simulink model "model6"  (R2022a)
settings: Solver=FixedStepAuto  StartTime=0.0  StopTime=200  FixedStep=1  RelTol=1e-3
values from neighbouring files (symbols this model uses):
  testMap = [0  0  0; 0  99  0; 0  0  0]    [aufgabe2.mat]
settings Model: Creator=JadKHaddad  LastModifiedBy=JadKHaddad

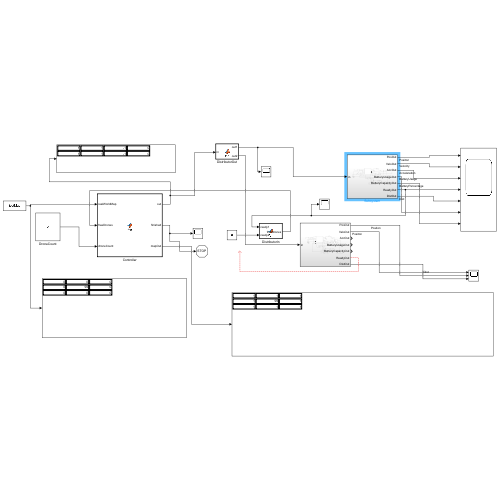
[thumbnail: Simulink's stored preview of the top-level diagram]
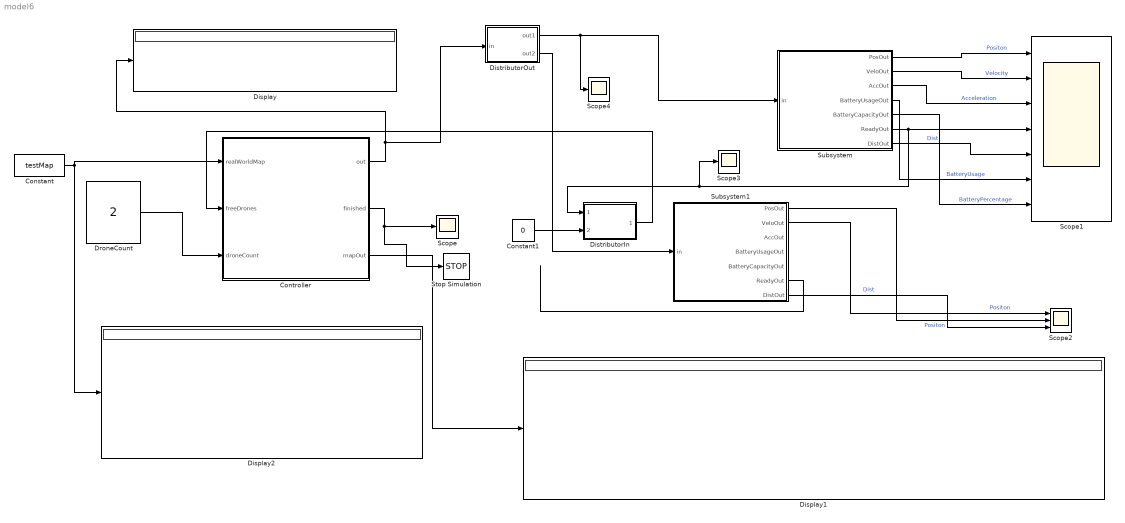
== system model6 ==
  Constant : Constant  Value=testMap  VectorParams1D=off
  Constant1 : Constant  Value=0
  Controller : MATLAB Function  TreatAsAtomicUnit=on
  Display : Display
  Display1 : Display
  Display2 : Display
  DistributorIn : MATLAB Function  TreatAsAtomicUnit=on
  DistributorOut : MATLAB Function  TreatAsAtomicUnit=on
  DroneCount : Constant  Value=2
  Scope : Scope
  Scope1 : Scope  NumInputPorts=7
  Scope2 : Scope  NumInputPorts=3
  Scope3 : Scope
  Scope4 : Scope
  Stop Simulation : Stop
  Subsystem : Subsystem
  Subsystem1 : Subsystem
  wires:
  Subsystem/3(AccOut) -> Scope1/3  "Acceleration"
  Subsystem/1(PosOut) -> Scope1/1  "Positon"
  Subsystem/4(BatteryUsageOut) -> Scope1/6  "BatteryUsage"
  Subsystem/2(VeloOut) -> Scope1/2  "Velocity"
  Subsystem/5(BatteryCapacityOut) -> Scope1/7  "BatteryPercentage"
  Subsystem/6(ReadyOut) -> Scope3/1, DistributorIn/1(ready1), Scope1/4
  Subsystem/7(DistOut) -> Scope1/5  "Dist"
  Controller/2(finished) -> Stop Simulation/1, Scope/1
  Constant/1 -> Display2/1, Controller/1(realWorldMap)
  DroneCount/1 -> Controller/3(droneCount)
  Controller/1(out) -> DistributorOut/1(in), Display/1
  DistributorIn/1(freeDrones) -> Controller/2(freeDrones)
  DistributorOut/1(out1) -> Scope4/1, Subsystem/1(in)
  Controller/3(mapOut) -> Display1/1
  DistributorOut/2(out2) -> Subsystem1/1(in)
  Subsystem1/1(PosOut) -> Scope2/2  "Positon"
  Subsystem1/6(ReadyOut) -> ?
  Subsystem1/7(DistOut) -> Scope2/3  "Dist"
  Subsystem1/2(VeloOut) -> Scope2/1  "Positon"
  Constant1/1 -> DistributorIn/2(ready2)

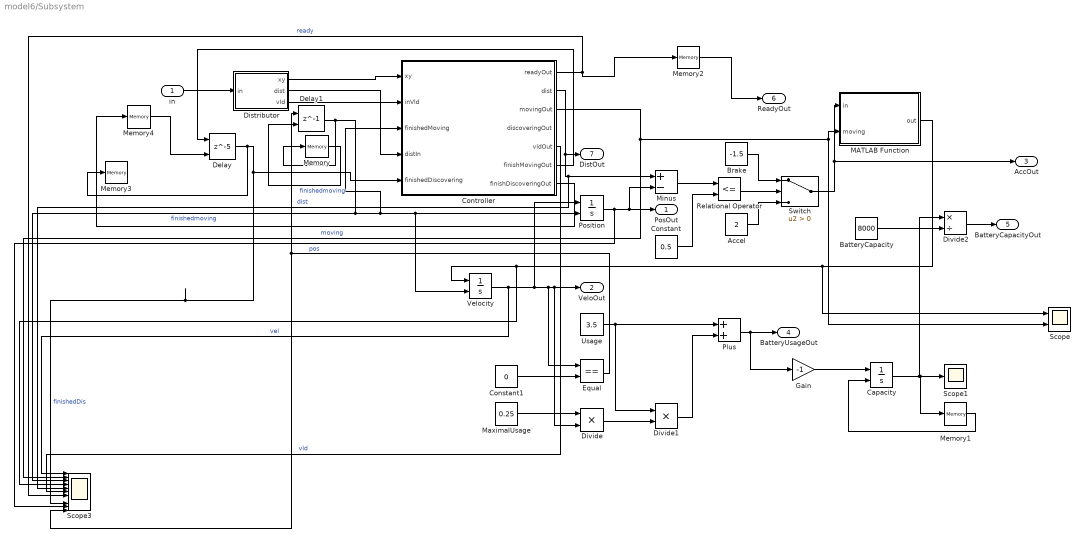
== system model6/Subsystem ==
  in : Inport
  Accel : Constant  Value=2
  BatteryCapacity : Constant  Value=8000
  Brake : Constant  Value=-1.5
  Capacity : Integrator  ExternalReset=rising  InitialCondition=8000  LowerSaturationLimit=0
  Constant : Constant  Value=0.5
  Constant1 : Constant  Value=0
  Controller : MATLAB Function  TreatAsAtomicUnit=on
  Delay : Delay  DelayLength=5  InitialCondition=0  ExternalReset=Rising
      settings: InputPortMap=u0,r5
  Delay1 : Delay  DelayLength=1  ExternalReset=Rising
      settings: InputPortMap=u0,r5
  Distributor : MATLAB Function  TreatAsAtomicUnit=on
  Divide : Product  Inputs=**  RndMeth=Round
  Divide1 : Product  Inputs=**
  Divide2 : Product  Inputs=*/
  Equal : RelationalOperator  Operator===  OutDataTypeStr=boolean  RndMeth=Simplest  InputSameDT=off
  Gain : Gain  Gain=-1
  MATLAB Function : MATLAB Function  TreatAsAtomicUnit=on
  MaximalUsage : Constant  Value=0.25
  Memory : Memory  InheritSampleTime=on
  Memory{1..4} (4 alike) : Memory
  Minus : Sum  Inputs=+-
  Plus : Sum
  Position : Integrator  ExternalReset=rising
  Relational Operator : RelationalOperator  Operator=<=  OutDataTypeStr=boolean  RndMeth=Simplest  InputSameDT=off
  Scope : Scope  NumInputPorts=2
  Scope1 : Scope
  Scope3 : Scope  NumInputPorts=11
  Switch : Switch  Criteria=u2 > Threshold  SaturateOnIntegerOverflow=off  InputSameDT=off
  Usage : Constant  Value=3.5
  Velocity : Integrator  ExternalReset=rising  LimitOutput=on  UpperSaturationLimit=1  LowerSaturationLimit=0
  PosOut : Outport
  VeloOut : Outport  Port=2
  AccOut : Outport  Port=3
  BatteryUsageOut : Outport  Port=4
  BatteryCapacityOut : Outport  Port=5
  ReadyOut : Outport  Port=6
  DistOut : Outport  Port=7
  wires:
  Controller/1(readyOut) -> Memory2/1, Scope3/7  "ready"
  Distributor/1(xy) -> Controller/1(xy)
  Distributor/3(vld) -> Controller/2(inVld)
  Switch/1 -> MATLAB Function/1(in), AccOut/1
  Plus/1 -> Gain/1, BatteryUsageOut/1
  Accel/1 -> Switch/3
  Divide2/1 -> BatteryCapacityOut/1
  Divide/1 -> Divide1/2
  Memory1/1 -> Capacity/2
  Distributor/2(dist) -> Controller/4(distIn)
  Usage/1 -> Plus/1, Divide1/1
  BatteryCapacity/1 -> Divide2/2
  Capacity/1 -> Memory1/1, Scope1/1, Divide2/1
  Gain/1 -> Capacity/1
  Divide1/1 -> Plus/2
  Minus/1 -> Relational Operator/1
  Position/1 -> Scope3/10, Minus/2, PosOut/1  "pos"
  Brake/1 -> Switch/1
  Constant1/1 -> Equal/2
  Relational Operator/1 -> Switch/2
  MaximalUsage/1 -> Divide/1
  Constant/1 -> Relational Operator/2
  Controller/2(dist) -> Minus/1, Scope3/5, DistOut/1  "dist"
  Velocity/1 -> Scope3/1, VeloOut/1, Divide/2, Equal/1, Position/1  "vel"
  Delay1/1 -> Memory/1, Scope3/3, Controller/3(finishedMoving), Velocity/2, Position/2  "finishedmoving"
  in/1 -> Distributor/1(in)
  Memory2/1 -> ReadyOut/1
  MATLAB Function/1(out) -> Scope/1, Scope3/4, Velocity/1
  Equal/1 -> Delay1/1, Scope3/11
  Delay/1 -> Memory3/1, Controller/5(finishedDiscovering), Scope3/9  "finishedDis"
  Controller/3(movingOut) -> Scope3/2, MATLAB Function/2(moving), Scope/2  "moving"
  Controller/5(vldOut) -> Scope3/6  "vld"
  Memory/1 -> Delay1/2  "finishedmoving"
  Controller/7(finishDiscoveringOut) -> Memory4/1
  Memory4/1 -> Delay/2
  Controller/6(finishMovingOut) -> Delay/1

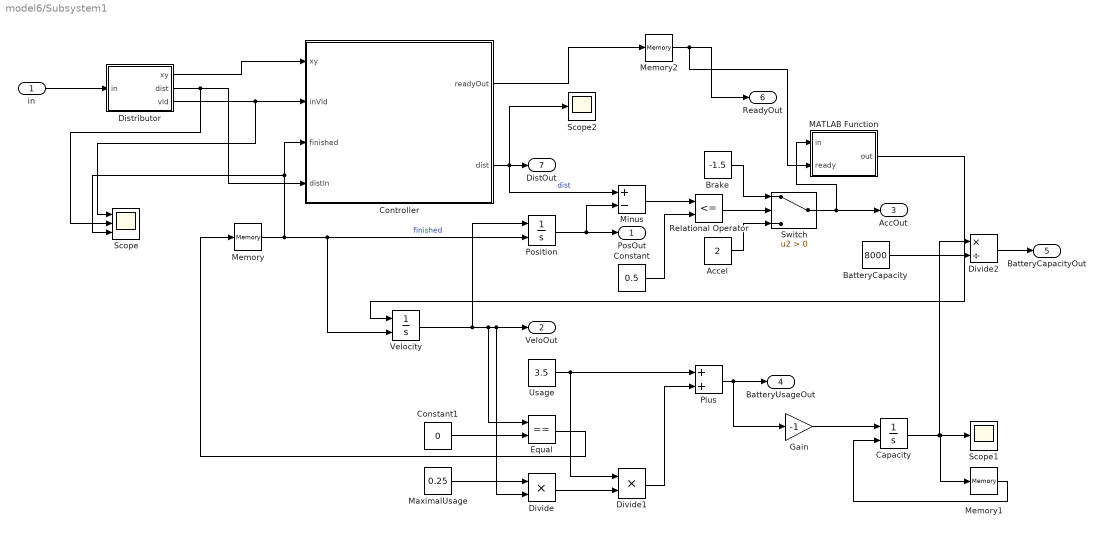
== system model6/Subsystem1 ==
  in : Inport
  Accel : Constant  Value=2
  BatteryCapacity : Constant  Value=8000
  Brake : Constant  Value=-1.5
  Capacity : Integrator  ExternalReset=rising  InitialCondition=8000  LowerSaturationLimit=0
  Constant : Constant  Value=0.5
  Constant1 : Constant  Value=0
  Controller : MATLAB Function  TreatAsAtomicUnit=on
  Distributor : MATLAB Function  TreatAsAtomicUnit=on
  Divide : Product  Inputs=**  RndMeth=Round
  Divide1 : Product  Inputs=**
  Divide2 : Product  Inputs=*/
  Equal : RelationalOperator  Operator===  OutDataTypeStr=boolean  RndMeth=Simplest  InputSameDT=off
  Gain : Gain  Gain=-1
  MATLAB Function : MATLAB Function  TreatAsAtomicUnit=on
  MaximalUsage : Constant  Value=0.25
  Memory : Memory
  Memory1 : Memory
  Memory2 : Memory
  Minus : Sum  Inputs=+-
  Plus : Sum
  Position : Integrator  ExternalReset=rising
  Relational Operator : RelationalOperator  Operator=<=  OutDataTypeStr=boolean  RndMeth=Simplest  InputSameDT=off
  Scope : Scope  NumInputPorts=3
  Scope1 : Scope
  Scope2 : Scope
  Switch : Switch  Criteria=u2 > Threshold  SaturateOnIntegerOverflow=off  InputSameDT=off
  Usage : Constant  Value=3.5
  Velocity : Integrator  ExternalReset=rising  LimitOutput=on  UpperSaturationLimit=1  LowerSaturationLimit=0
  PosOut : Outport
  VeloOut : Outport  Port=2
  AccOut : Outport  Port=3
  BatteryUsageOut : Outport  Port=4
  BatteryCapacityOut : Outport  Port=5
  ReadyOut : Outport  Port=6
  DistOut : Outport  Port=7
  wires:
  Controller/1(readyOut) -> Memory2/1
  Distributor/1(xy) -> Controller/1(xy)
  Distributor/3(vld) -> Scope/1, Controller/2(inVld)
  Switch/1 -> MATLAB Function/1(in), AccOut/1
  Plus/1 -> Gain/1, BatteryUsageOut/1
  Accel/1 -> Switch/3
  Divide2/1 -> BatteryCapacityOut/1
  Divide/1 -> Divide1/2
  Memory1/1 -> Capacity/2
  Distributor/2(dist) -> Scope/2, Controller/4(distIn)
  Usage/1 -> Plus/1, Divide1/1
  BatteryCapacity/1 -> Divide2/2
  Capacity/1 -> Memory1/1, Scope1/1, Divide2/1
  Gain/1 -> Capacity/1
  Divide1/1 -> Plus/2
  Minus/1 -> Relational Operator/1
  Position/1 -> Minus/2, PosOut/1
  Equal/1 -> Memory/1
  Brake/1 -> Switch/1
  Constant1/1 -> Equal/2
  Relational Operator/1 -> Switch/2
  MaximalUsage/1 -> Divide/1
  Constant/1 -> Relational Operator/2
  Controller/2(dist) -> Scope2/1, Minus/1, DistOut/1  "dist"
  Velocity/1 -> VeloOut/1, Divide/2, Equal/1, Position/1
  Memory/1 -> Velocity/2, Position/2, Controller/3(finished), Scope/3  "finished"
  in/1 -> Distributor/1(in)
  Memory2/1 -> MATLAB Function/2(ready), ReadyOut/1
  MATLAB Function/1(out) -> Velocity/1

== matlab function model6/Subsystem/Distributor ==
  data: in input; xy output; dist output; vld output
function [xy,dist,vld] = fcn(in)
xy = [-1 -1];
dist = -1;
vld = 0;

xy = [in(1) in(2)];
dist = in(3);
vld = in(4);
end

== matlab function model6/Controller ==
  data: realWorldMap input; out output; finished output; freeDrones input; droneCount input; mapOut output
function [out, finished, mapOut] = fcn(realWorldMap, freeDrones, droneCount)
    disp("-------------------------------");
%     i = 1;
%     while i <= droneCount
%        droneIsFree = freeDrones(1, i);
%        fprintf("Drone: [%d] ready: %d\n", int8(i), int8(droneIsFree));
%        i = i +1;
%     end

    persistent index
    persistent indexLimit
    persistent path
    persistent lastXY
    persistent workingDronesCount
    persistent cameBackDronesCount
    persistent map
    persistent workingDrones
    persistent inTermMode
    
    if isempty(inTermMode)
        inTermMode = 0;
    end

    if isempty(workingDrones)
        workingDrones = zeros(droneCount);
    end
    if isempty(workingDronesCount)
        workingDronesCount = 0;
    end
    if isempty(cameBackDronesCount)
        cameBackDronesCount = 0;
    end
    if isempty(index)
        index = 1;
    end
    if isempty(indexLimit)
        indexLimit = 2;
    end
    if isempty(path)
        path = ones(length(realWorldMap)*length(realWorldMap),2);
    end
    if isempty(lastXY)
        lastXY = ones(droneCount, 2);
        lastXY = -1 * lastXY;
    end
    if isempty(map)
        map = zeros(length(realWorldMap), length(realWorldMap));
    end

    function indexDist = getIndexAndDistOfAFreeDrone(dest)
        DIndex = -1;
        minDist = -1;
        i = 1;
        while(i <= droneCount)
            if(freeDrones(i) == 1)
                source = lastXY(i,:);
                if source(1) == -2
                    i = i + 1;
                    continue
                end
                if(source(1) == -1)
                    source(1) = 1;
                end
                if(source(2) == -1)
                    source(2) = 1;
                end
                dist = minDistanceSimulink(map, source(1), source(2), dest(1), dest(2));
                if(minDist == -1 && dist ~= -1) || (minDist ~= -1 && dist ~= -1 && dist < minDist)
                    minDist = dist;
                    DIndex = i;
                end
            end
            i = i + 1;
        end
        indexDist = [DIndex minDist];
    end

    finished = 0;
    mapOut = map;

    %out = [xy(1) xy(2) dist vld];
    out = ones(2, 4);
    i = 1;
    while (i <= droneCount)
       out(i,:) = [1 1 -1 0];
       i = i + 1;
    end

    %sink
    if cameBackDronesCount >= droneCount
        finished = 1;
        fprintf("All drones came back. Terminating.");
        return
    end
    i = 1;
    while i <= droneCount
        x = lastXY(i, 1);
        y = lastXY(i, 2);
        droneIsFree = freeDrones(1, i);
        if droneIsFree == 1 && x == -2
            cameBackDronesCount = cameBackDronesCount + 1;
            fprintf("Drone [%d] came back\n", int8(i));
            lastXY(i,:) = [-3 -3];
            i = i + 1;
            continue
        end
        if droneIsFree == 1 && x ~= -1 && x ~= -2 && x ~= -3 && workingDrones(i) == 1
            %update path
            fprintf("Drone [%d] is now ready\n", int8(i));
            workingDrones(i) = 0;
            workingDronesCount = workingDronesCount - 1;
            map(x,y) = 3;
            if realWorldMap(x,y) == 0
                if x + 1 <= length(realWorldMap) && map(x + 1, y) == 0
                    if realWorldMap(x + 1, y) == 0
                        newRow = [x+1 y];
                        map(x+1,y) = -1;
                        path(indexLimit,:) = newRow;
                        indexLimit = indexLimit + 1;
                    else
                        map(x+1,y) = 99;
                    end
                end
                
                if y + 1 <= length(realWorldMap) && map(x, y + 1) == 0
                    if realWorldMap(x, y + 1) == 0
                        newRow = [x y+1];
                        map(x,y+1) = -1;
                        path(indexLimit,:) = newRow;
                        indexLimit = indexLimit + 1;
                    else
                        map(x, y + 1) = 99;
                    end
                end
                
                if x - 1 >= 1 && map(x - 1, y) == 0 
                    if realWorldMap(x - 1, y) == 0 
                        newRow = [x-1 y];
                        map(x-1,y) = -1;
                        path(indexLimit-1,:) = newRow;
                        indexLimit = indexLimit + 1;
                    else
                        map(x - 1, y) = 99;
                    end
                end
                
                if y - 1 >= 1 && map(x, y-1) == 0
                    if realWorldMap(x, y-1) == 0
                        newRow = [x y-1];
                        map(x,y-1) = -1;
                        path(indexLimit,:) = newRow;
                        indexLimit = indexLimit + 1;
                    else
                        map(x, y-1) = 99;
                    end
                end
            end
        end
        i = i + 1;
    end


    if index >= indexLimit
        if workingDronesCount == 0
            if inTermMode == 0
                disp("Entering termination modus");
                inTermMode = 1;
            end
            droneIndex = 1;
            while droneIndex <= droneCount
                droneLocation = lastXY(droneIndex,:);
                if droneLocation(1) == -1
                    fprintf("Drone [%d] is already at start location\n", int8(droneIndex));
                    lastXY(droneIndex, :) = [-3 -3];
                    cameBackDronesCount = cameBackDronesCount + 1;
                    droneIndex = droneIndex + 1;
                    continue
                end
                if droneLocation(1) == -3 || droneLocation(1) == -2
                    droneIndex = droneIndex + 1;
                    continue
                end
                droneIsFree = freeDrones(1, droneIndex);
                if droneIsFree == 1
                    dist = minDistanceSimulink(map, droneLocation(1), droneLocation(2), 1, 1);
                    out(droneIndex,1) = -2;
                    out(droneIndex,2) = -2;
                    out(droneIndex,3) = dist;
                    out(droneIndex,4) = 1;
                    fprintf("Calling drone [%d] back from(%d, %d) with distance [%d]\n", int8(droneIndex), int8(lastXY(droneIndex,1)), int8(lastXY(droneIndex,2)), int8(dist));
    
                    map(droneLocation(1), droneLocation(2)) = 1;
                    lastXY(droneIndex,:) = [-2 -2];
                end
                droneIndex = droneIndex + 1;
            end
        end

    else
        dest = path(index,:);
        indexDist = getIndexAndDistOfAFreeDrone(dest);
        droneIndex = indexDist(1);
        dist = indexDist(2);
        %X = sprintf('index: %f, dest; %f %f dist %f',droneIndex,dest(1), dest(2), dist);
        %disp(X);
        if droneIndex > -1 && dist > -1
            out(droneIndex,1) = dest(1);
            out(droneIndex,2) = dest(2);
            out(droneIndex,3) = dist;
            out(droneIndex,4) = 1;
            fprintf("Sending drone [%d] from(%d, %d) to (%d, %d) with distance [%d]\n", int8(droneIndex), int8(lastXY(droneIndex,1)), int8(lastXY(droneIndex,2)), int8(dest(1)), int8(dest(2)), int8(dist));
            workingDronesCount = workingDronesCount + 1;
            workingDrones(droneIndex) = 1;
            if lastXY(droneIndex,1) ~= -1
                if map(lastXY(droneIndex,1), lastXY(droneIndex,2)) == 3
                    map(lastXY(droneIndex,1), lastXY(droneIndex,2)) = 1;
                end
            end
            map(dest(1),dest(2)) = 2;
            lastXY(droneIndex,:) = dest;
            index = index + 1;
        end
    end
end

== matlab function model6/Subsystem/Controller ==
  settings: updateMethod=DISCRETE
  data: xy input; readyOut output; inVld input; finishedMoving input; dist output; distIn input; finishedDiscovering input; movingOut output; discoveringOut output; vldOut output; finishMovingOut output; finishDiscoveringOut output
function [readyOut, dist, movingOut, discoveringOut, vldOut, finishMovingOut, finishDiscoveringOut] = fcn(xy, inVld, finishedMoving, distIn, finishedDiscovering)

persistent distance
persistent ready
persistent moving
persistent ignoreMoving
persistent ignoreDiscovering
persistent discovering

if isempty(ignoreMoving)
    ignoreMoving = 1;
end
if isempty(ignoreDiscovering)
    ignoreDiscovering = 1;
end
if isempty(ready)
    ready = 1;
end

if isempty(moving)
    moving = 0;
end

if isempty(discovering)
    discovering = 0;
end
if isempty(distance)
    distance = -1;
end

finishMovingOut = 0;
finishDiscoveringOut = 0;

if finishedMoving == 1 && ignoreMoving == 0
    disp("finish move sig is on");
    if moving == 1
        moving = 0;
        finishMovingOut = 1;
        discovering = 1;
        disp("finished moving");
        ignoreMoving = 1;
        ignoreDiscovering = 0;
    end
    
end

if finishedDiscovering == 1 && ignoreDiscovering == 0
    disp("finish discover sig is on");
    if discovering == 1
        ignoreDiscovering = 1;
        discovering = 0;
        finishDiscoveringOut = 1;
        disp("finished discovering");
    end
    
end

if inVld == 1 && ready == 1
    ready = 0;
    distance = distIn;
    moving = 1;
    ignoreMoving = 0;
    discovering = 0;
end

if discovering == 1 || moving == 1
    ready = 0;
end

if discovering == 0 && moving == 0
    ready = 1;
end

if ready == 1
    disp("ready")
end
if moving == 1
    disp("moving")
end
if discovering
    disp("discovering")
end

dist = distance;
discoveringOut = discovering;
movingOut = moving;
readyOut = ready;
vldOut = inVld;

== matlab function model6/Subsystem1/Controller ==
  settings: updateMethod=DISCRETE
  data: xy input; readyOut output; inVld input; finished input; dist output; distIn input
function [readyOut, dist] = fcn(xy, inVld, finished, distIn)

persistent distance

if isempty(distance)
    distance = -1;
end
dist = distance;
ready = 0;

if finished == 1
    ready = 1;
end

if inVld == 1 && ready == 1
    ready = 0;
    distance = distIn;
    dist = distIn;
end


readyOut = ready;

== matlab function model6/Subsystem1/Distributor ==
  data: in input; xy output; dist output; vld output
function [xy,dist,vld] = fcn(in)
xy = [-1 -1];
dist = -1;
vld = 0;

xy = [in(1) in(2)];
dist = in(3);
vld = in(4);
end

== matlab function model6/DistributorOut ==
  data: in input; out1 output; out2 output
function [out1, out2] = fcn(in)
    out1 = [1 1 -1 0];
    out2 = [1 1 -1 0];
    
    out1 = in(1,:);
    out2 = in(2,:);
end

== matlab function model6/DistributorIn ==
  data: ready1 input; freeDrones output; ready2 input
function freeDrones = fcn(ready1, ready2)
    freeDrones = [ready1 ready2];
end

== matlab function model6/Subsystem/MATLAB Function ==
  data: in input; out output; moving input
function out = fcn(in, moving)
    out = 0;
    if moving == 1
        out = in;
    end

== matlab function model6/Subsystem1/MATLAB Function ==
  data: in input; out output; ready input
function out = fcn(in, ready)
    out = 0;
    if ready == 0
        out = in;
    end
